simulink library "wcdma_lib"  (Simulink 6.0)
settings: Solver=ode45  SolverMode=SingleTasking  StartTime=0.0  StopTime=10.0  RelTol=1e-3
values from neighbouring files (symbols this model uses):
  allocationssc = [1 1 1 1 1 1 1 1 1 1 1 1 ... (960 elements, 64x15)]    [wcdma_allocationssc.mat]
  crcSize = str2num(Vals{idxCrcSize})    [wcdma_initmaskphlayer.m]    (also in wcdma_loadinitmuxandcoding.m = [16 12]; wcdma_loadinitphlayer.m = [16 12])
  errorCorr = (errorCorr>2)*2 + (errorCorr<3).*errorCorr    [wcdma_initmaskphlayer.m]    (also in wcdma_loadinitmuxandcoding.m = [2 2]; wcdma_loadinitphlayer.m = [2 2])
  i = [1:2:numSamp-1]'    [cdma2000_inttable.m]
  numBitsCodeWord = cond.*Zmin + not(cond).*numBitsCodeWord    [wcdma_concseg.m]    (also in wcdma_loadinitmuxandcoding.m = [260 122])
  numBitsFirstInt = numBitsRM + deltaNimax    [wcdma_initmaskphlayer.m]    (also in wcdma_loadinitmuxandcoding.m = [686 308])
  numBitsRF = numBitsFirstInt./(tti/10)    [wcdma_initmaskphlayer.m]    (also in wcdma_loadinitmuxandcoding.m = [343 77]; wcdma_loadinitphlayer.m = [343 77])
  numBitsTrCh = (trBlkSize+crcSize)*diag(numTrBlks)    [wcdma_concseg.m]    (also in wcdma_loadinitmuxandcoding.m = [260 112])
  numCodeWords = ceil(numBitsTrCh./Zmax(errorCorr+1))    [wcdma_concseg.m]    (also in wcdma_loadinitmuxandcoding.m = [1 1])
  numPadBits = (numBitsCodeWord.*numCodeWords)-numBitsTrCh    [wcdma_concseg.m]    (also in wcdma_loadinitmuxandcoding.m = [0 0])
  numPhCH = str2num(Vals{idxNumPhCH})    [wcdma_initmaskphlayer.m]    (also in wcdma_loadinitmuxandcoding.m = 1; wcdma_loadinitphlayer.m = 1)
  numTrBlks = trBlkSetSize./trBlkSize    [wcdma_concseg.m]    (also in wcdma_initmaskphlayer.m; wcdma_loadinitmuxandcoding.m = [1 1]; wcdma_loadinitphlayer.m = [1 1])
  overSampling = str2num(Vals{idxOverSampling})    [wcdma_initmaskphlayer.m]    (also in wcdma_initmaskspreadandmod.m; wcdma_loadinitphlayer.m = 8; wcdma_loadinitspreadandmod.m = 8)
  powerVector = str2num(Vals{idxPowerVector})    [wcdma_initmaskphlayer.m]    (also in wcdma_initmaskspreadandmod.m; wcdma_loadinitphlayer.m = [-5.5 -10 -15 -12 -12]; wcdma_loadinitspreadandmod.m = [-5.5 -10 -15 -12 -12])
  sprdFactor = wcdma_slotformattable(slotFormat+1,2)    [wcdma_checkparamstxant.m]    (also in wcdma_initmaskphlayer.m = slotformattable(slotFormat+1,2); wcdma_initmaskspreadandmod.m = slotformattable(slotFormat+1,2); wcdma_loadinitphlayer.m = 128; wcdma_loadinitspreadandmod.m = 128)
  tti = str2num(Vals{idxTti})    [wcdma_initmaskphlayer.m]    (also in wcdma_loadinitmuxandcoding.m = [20 40]; wcdma_loadinitphlayer.m = [20 40])
undefined symbols (not defined in the file or in its folder): hadamard, numSymbOut
libraries: wcdma_lib x122, dspsrcs4 x39, dspsigops x30, commseqgen2 x24, dspindex x20, dspbuff3 x19, dspmathops x16, simulink x10, dspsigattribs x7, commutil2 x6, dspmtrx3 x6, commblkintrlv2 x6
(part 3 of 3)

== system wcdma_lib/Wcdma Multiplexing and Channel Coding/Wcdma Tx  Channel Coding Scheme ==
  note: Wcdma Physical Channel TX Error Correction
  note: CRC
      | Calculation
  note: TrBlk Concat/
      | Code Blk Segm
  note: Channel
      | Coding
  note: 1st
      | Interleaver
  note: Rate
      | Matching
  note: Radio Frame
      | Segmentation
  TrChIn1 : Inport  LatchInput=off
  TrChIn2 : Inport  Port=2  LatchInput=off
  1st Interleaver : wcdma_lib/Wcdma Multiplexing and Channel Coding/1st Interleaver
  CRC Calculation : wcdma_lib/Wcdma Multiplexing and Channel Coding/CRC Calculation
  Channel Encoding : wcdma_lib/Wcdma Multiplexing and Channel Coding/Channel Encoding
  Radio Frame  Segmentation : wcdma_lib/Wcdma Multiplexing and Channel Coding/Radio Frame  Segmentation
  Rate Matching : wcdma_lib/Wcdma Multiplexing and Channel Coding/Rate Matching
  TrBlk Concatenat Code Blk Segment : wcdma_lib/Wcdma Multiplexing and Channel Coding/TrBlk Concatenat Code Blk Segment  numBitsTrCh=numBitsTrCh  numPadBits=numPadBits  numBitsCodeWord=numBitsCodeWord
  background6 : Subsystem  EnableExecutionContextPropagation=on
      mask Display: disp('')
  CCTrChOut1 : Outport
  wires:
  CRC Calculation/1 -> TrBlk Concatenat Code Blk Segment/1  "dtch"
  CRC Calculation/2 -> TrBlk Concatenat Code Blk Segment/2  "dcch"
  TrBlk Concatenat Code Blk Segment/1 -> Channel Encoding/1  "dtch"
  TrBlk Concatenat Code Blk Segment/2 -> Channel Encoding/2  "dcch"
  Channel Encoding/1 -> Rate Matching/1  "dtch"
  Channel Encoding/2 -> Rate Matching/2  "dcch"
  Rate Matching/1 -> 1st Interleaver/1  "dtch"
  Rate Matching/2 -> 1st Interleaver/2  "dcch"
  TrChIn1/1 -> CRC Calculation/1  "dtch"
  TrChIn2/1 -> CRC Calculation/2  "dcch"
  1st Interleaver/1 -> Radio Frame  Segmentation/1  "dtch"
  1st Interleaver/2 -> Radio Frame  Segmentation/2  "dcch"
  Radio Frame  Segmentation/1 -> CCTrChOut1/1  "cctrch"

== system wcdma_lib/Wcdma Sources/Channel Generator ==
  "Complex Unipolar to Bipolar " : wcdma_lib/Wcdma Common/Complex Unipolar to Bipolar   M=2  polarity=Negative
  Deinterlacer : commsequence2/Deinterlacer
  Delay : dspsigops/Delay  dly_unit=Samples  delay=initDelay  ic_detail=off  dif_ic_for_ch=off  dif_ic_for_dly=off  ic=0  reset_popup=None
  Gain : Gain  Gain=1/sqrt(2)  SaturateOnIntegerOverflow=on
  Random-Integer Generator : commrandsrc2/Random Integer Generator  mul=2  seed=rndSeed  Ts=st/2  frameBased=on  sampPerFrame=2*numSymbOut  orient=off
  Real-Imag to Complex : RealImagToComplex
  cChannel : Outport
  wires:
  Deinterlacer/2 -> Real-Imag to Complex/2
  Deinterlacer/1 -> Real-Imag to Complex/1
  "Complex Unipolar to Bipolar "/1 -> Gain/1
  Real-Imag to Complex/1 -> "Complex Unipolar to Bipolar "/1
  Gain/1 -> Delay/1
  Random-Integer Generator/1 -> Deinterlacer/1
  Delay/1 -> cChannel/1

== system wcdma_lib/Wcdma Sources/P-CPICH Generator ==
  "Complex Unipolar to Bipolar " : wcdma_lib/Wcdma Common/Complex Unipolar to Bipolar   M=2  polarity=Negative
  DSP Constant : dspsrcs4/DSP Constant  Value=ones(2*numSymbOut,1)  InterpretAs1D=off  SampleMode=Discrete  Ts=numSymbOut*st  FramebasedOutput=on
  Deinterlacer : commsequence2/Deinterlacer
  Gain : Gain  Gain=1/sqrt(2)  SaturateOnIntegerOverflow=on
  Real-Imag to Complex : RealImagToComplex
  cP-CPICH : Outport
  wires:
  Gain/1 -> cP-CPICH/1
  "Complex Unipolar to Bipolar "/1 -> Gain/1
  DSP Constant/1 -> Deinterlacer/1
  Deinterlacer/1 -> Real-Imag to Complex/1
  Deinterlacer/2 -> Real-Imag to Complex/2
  Real-Imag to Complex/1 -> "Complex Unipolar to Bipolar "/1

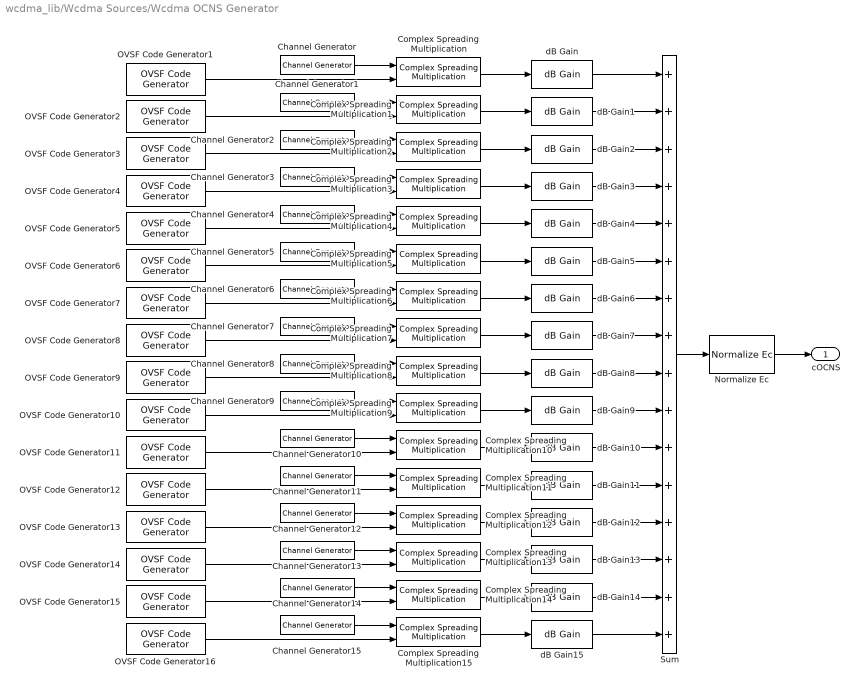
== system wcdma_lib/Wcdma Sources/Wcdma OCNS Generator ==
  Channel Generator : wcdma_lib/Wcdma Sources/Channel Generator  rndSeed=8686  initDelay=86  numSymbOut=numSymbOut  st=1/15e3
  Channel Generator1 : wcdma_lib/Wcdma Sources/Channel Generator  rndSeed=134134  initDelay=134  numSymbOut=numSymbOut  st=1/15e3
  Channel Generator10 : wcdma_lib/Wcdma Sources/Channel Generator  rndSeed=3030  initDelay=30  numSymbOut=numSymbOut  st=1/15e3
  Channel Generator11 : wcdma_lib/Wcdma Sources/Channel Generator  rndSeed=1818  initDelay=18  numSymbOut=numSymbOut  st=1/15e3
  Channel Generator12 : wcdma_lib/Wcdma Sources/Channel Generator  rndSeed=3030  initDelay=30  numSymbOut=numSymbOut  st=1/15e3
  Channel Generator13 : wcdma_lib/Wcdma Sources/Channel Generator  rndSeed=6161  initDelay=61  numSymbOut=numSymbOut  st=1/15e3
  Channel Generator14 : wcdma_lib/Wcdma Sources/Channel Generator  rndSeed=128128  initDelay=128  numSymbOut=numSymbOut  st=1/15e3
  Channel Generator15 : wcdma_lib/Wcdma Sources/Channel Generator  rndSeed=143143  initDelay=143  numSymbOut=numSymbOut  st=1/15e3
  Channel Generator2 : wcdma_lib/Wcdma Sources/Channel Generator  rndSeed=5252  initDelay=52  numSymbOut=numSymbOut  st=1/15e3
  Channel Generator3 : wcdma_lib/Wcdma Sources/Channel Generator  rndSeed=4545  initDelay=45  numSymbOut=numSymbOut  st=1/15e3
  Channel Generator4 : wcdma_lib/Wcdma Sources/Channel Generator  rndSeed=143143  initDelay=143  numSymbOut=numSymbOut  st=1/15e3
  Channel Generator5 : wcdma_lib/Wcdma Sources/Channel Generator  rndSeed=112112  initDelay=112  numSymbOut=numSymbOut  st=1/15e3
  Channel Generator6 : wcdma_lib/Wcdma Sources/Channel Generator  rndSeed=5959  initDelay=59  numSymbOut=numSymbOut  st=1/15e3
  Channel Generator7 : wcdma_lib/Wcdma Sources/Channel Generator  rndSeed=2323  initDelay=23  numSymbOut=numSymbOut  st=1/15e3
  Channel Generator8 : wcdma_lib/Wcdma Sources/Channel Generator  rndSeed=11  initDelay=1  numSymbOut=numSymbOut  st=1/15e3
  Channel Generator9 : wcdma_lib/Wcdma Sources/Channel Generator  rndSeed=8888  initDelay=88  numSymbOut=numSymbOut  st=1/15e3
  Complex Spreading Multiplication{,1..15} (16 alike) : wcdma_lib/Wcdma BS Transmitter/Complex Spreading Multiplication  sprdFactor=sprdFactor
  Normalize Ec : wcdma_lib/Wcdma Common/Normalize Ec
  OVSF Code Generator1 : commseqgen2/OVSF Code Generator  spreadFact=256  index=2  ts=1/15e3  frameBased=on  sampPerFrame=numChipsOut
  OVSF Code Generator10 : commseqgen2/OVSF Code Generator  spreadFact=256  index=69  ts=1/15e3  frameBased=on  sampPerFrame=numChipsOut
  OVSF Code Generator11 : commseqgen2/OVSF Code Generator  spreadFact=256  index=78  ts=1/15e3  frameBased=on  sampPerFrame=numChipsOut
  OVSF Code Generator12 : commseqgen2/OVSF Code Generator  spreadFact=256  index=85  ts=1/15e3  frameBased=on  sampPerFrame=numChipsOut
  OVSF Code Generator13 : commseqgen2/OVSF Code Generator  spreadFact=256  index=94  ts=1/15e3  frameBased=on  sampPerFrame=numChipsOut
  OVSF Code Generator14 : commseqgen2/OVSF Code Generator  spreadFact=256  index=125  ts=1/15e3  frameBased=on  sampPerFrame=numChipsOut
  OVSF Code Generator15 : commseqgen2/OVSF Code Generator  spreadFact=256  index=113  ts=1/15e3  frameBased=on  sampPerFrame=numChipsOut
  OVSF Code Generator16 : commseqgen2/OVSF Code Generator  spreadFact=256  index=119  ts=1/15e3  frameBased=on  sampPerFrame=numChipsOut
  OVSF Code Generator2 : commseqgen2/OVSF Code Generator  spreadFact=256  index=11  ts=1/15e3  frameBased=on  sampPerFrame=numChipsOut
  OVSF Code Generator3 : commseqgen2/OVSF Code Generator  spreadFact=256  index=17  ts=1/15e3  frameBased=on  sampPerFrame=numChipsOut
  OVSF Code Generator4 : commseqgen2/OVSF Code Generator  spreadFact=256  index=23  ts=1/15e3  frameBased=on  sampPerFrame=numChipsOut
  OVSF Code Generator5 : commseqgen2/OVSF Code Generator  spreadFact=256  index=31  ts=1/15e3  frameBased=on  sampPerFrame=numChipsOut
  OVSF Code Generator6 : commseqgen2/OVSF Code Generator  spreadFact=256  index=38  ts=1/15e3  frameBased=on  sampPerFrame=numChipsOut
  OVSF Code Generator7 : commseqgen2/OVSF Code Generator  spreadFact=256  index=47  ts=1/15e3  frameBased=on  sampPerFrame=numChipsOut
  OVSF Code Generator8 : commseqgen2/OVSF Code Generator  spreadFact=256  index=55  ts=1/15e3  frameBased=on  sampPerFrame=numChipsOut
  OVSF Code Generator9 : commseqgen2/OVSF Code Generator  spreadFact=256  index=62  ts=1/15e3  frameBased=on  sampPerFrame=numChipsOut
  Sum : Sum  Inputs=++++++++++++++++  SaturateOnIntegerOverflow=on  InputSameDT=on
  dB Gain : dspmathops/dB Gain  dB=-1  intype=Amplitude
  dB Gain1 : dspmathops/dB Gain  dB=-3  intype=Amplitude
  dB Gain10 : dspmathops/dB Gain  dB=-5  intype=Amplitude
  dB Gain11 : dspmathops/dB Gain  dB=-9  intype=Amplitude
  dB Gain12 : dspmathops/dB Gain  dB=-10  intype=Amplitude
  dB Gain13 : dspmathops/dB Gain  dB=-8  intype=Amplitude
  dB Gain14 : dspmathops/dB Gain  dB=-6  intype=Amplitude
  dB Gain15 : dspmathops/dB Gain  dB=0  intype=Amplitude
  dB Gain2 : dspmathops/dB Gain  dB=-3  intype=Amplitude
  dB Gain3 : dspmathops/dB Gain  dB=-5  intype=Amplitude
  dB Gain4 : dspmathops/dB Gain  dB=-2  intype=Amplitude
  dB Gain5 : dspmathops/dB Gain  dB=-4  intype=Amplitude
  dB Gain6 : dspmathops/dB Gain  dB=-8  intype=Amplitude
  dB Gain7 : dspmathops/dB Gain  dB=-7  intype=Amplitude
  dB Gain8 : dspmathops/dB Gain  dB=-4  intype=Amplitude
  dB Gain9 : dspmathops/dB Gain  dB=-6  intype=Amplitude
  cOCNS : Outport
  wires:
  Channel Generator/1 -> Complex Spreading Multiplication/1
  Channel Generator1/1 -> Complex Spreading Multiplication1/1
  Channel Generator2/1 -> Complex Spreading Multiplication2/1
  Channel Generator3/1 -> Complex Spreading Multiplication3/1
  Channel Generator4/1 -> Complex Spreading Multiplication4/1
  Channel Generator5/1 -> Complex Spreading Multiplication5/1
  Channel Generator6/1 -> Complex Spreading Multiplication6/1
  Channel Generator7/1 -> Complex Spreading Multiplication7/1
  Channel Generator8/1 -> Complex Spreading Multiplication8/1
  Channel Generator9/1 -> Complex Spreading Multiplication9/1
  Channel Generator10/1 -> Complex Spreading Multiplication10/1
  Channel Generator11/1 -> Complex Spreading Multiplication11/1
  Channel Generator12/1 -> Complex Spreading Multiplication12/1
  Channel Generator13/1 -> Complex Spreading Multiplication13/1
  Channel Generator14/1 -> Complex Spreading Multiplication14/1
  Channel Generator15/1 -> Complex Spreading Multiplication15/1
  OVSF Code Generator16/1 -> Complex Spreading Multiplication15/2
  OVSF Code Generator1/1 -> Complex Spreading Multiplication/2
  OVSF Code Generator2/1 -> Complex Spreading Multiplication1/2
  OVSF Code Generator3/1 -> Complex Spreading Multiplication2/2
  OVSF Code Generator4/1 -> Complex Spreading Multiplication3/2
  OVSF Code Generator5/1 -> Complex Spreading Multiplication4/2
  OVSF Code Generator6/1 -> Complex Spreading Multiplication5/2
  OVSF Code Generator7/1 -> Complex Spreading Multiplication6/2
  OVSF Code Generator8/1 -> Complex Spreading Multiplication7/2
  OVSF Code Generator9/1 -> Complex Spreading Multiplication8/2
  OVSF Code Generator10/1 -> Complex Spreading Multiplication9/2
  OVSF Code Generator11/1 -> Complex Spreading Multiplication10/2
  OVSF Code Generator12/1 -> Complex Spreading Multiplication11/2
  OVSF Code Generator13/1 -> Complex Spreading Multiplication12/2
  OVSF Code Generator14/1 -> Complex Spreading Multiplication13/2
  OVSF Code Generator15/1 -> Complex Spreading Multiplication14/2
  Complex Spreading Multiplication1/1 -> dB Gain1/1
  Complex Spreading Multiplication2/1 -> dB Gain2/1
  Complex Spreading Multiplication3/1 -> dB Gain3/1
  Complex Spreading Multiplication4/1 -> dB Gain4/1
  Complex Spreading Multiplication5/1 -> dB Gain5/1
  Complex Spreading Multiplication6/1 -> dB Gain6/1
  Complex Spreading Multiplication7/1 -> dB Gain7/1
  Complex Spreading Multiplication8/1 -> dB Gain8/1
  Complex Spreading Multiplication9/1 -> dB Gain9/1
  Complex Spreading Multiplication10/1 -> dB Gain10/1
  Complex Spreading Multiplication11/1 -> dB Gain11/1
  Complex Spreading Multiplication12/1 -> dB Gain12/1
  Complex Spreading Multiplication13/1 -> dB Gain13/1
  Complex Spreading Multiplication14/1 -> dB Gain14/1
  Complex Spreading Multiplication15/1 -> dB Gain15/1
  Sum/1 -> Normalize Ec/1
  dB Gain/1 -> Sum/1
  dB Gain1/1 -> Sum/2
  dB Gain2/1 -> Sum/3
  dB Gain3/1 -> Sum/4
  dB Gain4/1 -> Sum/5
  dB Gain5/1 -> Sum/6
  dB Gain6/1 -> Sum/7
  dB Gain7/1 -> Sum/8
  dB Gain8/1 -> Sum/9
  dB Gain9/1 -> Sum/10
  dB Gain10/1 -> Sum/11
  dB Gain11/1 -> Sum/12
  dB Gain12/1 -> Sum/13
  dB Gain13/1 -> Sum/14
  dB Gain14/1 -> Sum/15
  dB Gain15/1 -> Sum/16
  Complex Spreading Multiplication/1 -> dB Gain/1
  Normalize Ec/1 -> cOCNS/1

== system wcdma_lib/Wcdma Sources/Wcdma PSC Generator ==
  Frame Status Conversion : dspsigattribs/Frame Status Conversion  growRefPort=off  outframe=Frame-based
  Gain1 : Gain  Gain=1/sqrt(2)  SaturateOnIntegerOverflow=on
  Matrix Multiply : dspmtrx3/Matrix Multiply  numInputPorts=2  OptimizationLevel=None
  Pattern Repetition : dspsrcs4/DSP Constant  Value="[1 1 1 -1 -1 1 -1 -1  1 1 1 -1 1 -1 1 1]"  InterpretAs1D=off  SampleMode=Discrete  Ts=0.01/15  FramebasedOutput=on
  Real-Imag to Complex : RealImagToComplex
  Reshape : simulink3/Signals & Systems/Reshape  OutputDimensionality=Column vector  OutputDimensions=[1,1]
  Seq a : dspsrcs4/DSP Constant  Value=[1 1 1 1 1 1 -1 -1 1 -1 1 -1 1 -1 -1 1]'  InterpretAs1D=off  SampleMode=Discrete  Ts=0.01/15  FramebasedOutput=on
  PSC Code : Outport
  wires:
  Gain1/1 -> PSC Code/1
  Seq a/1 -> Matrix Multiply/1
  Pattern Repetition/1 -> Matrix Multiply/2
  Matrix Multiply/1 -> Reshape/1
  Real-Imag to Complex/1 -> Gain1/1
  Reshape/1 -> Frame Status Conversion/1
  Frame Status Conversion/1 -> Real-Imag to Complex/1, Real-Imag to Complex/2

== system wcdma_lib/Wcdma Sources/Wcdma Pilot Bits Generator ==
  Frame Status Conversion : dspsigattribs/Frame Status Conversion  growRefPort=off  outframe=Frame-based
  Integer to Bit Converter : commutil2/Integer to Bit Converter  nbits=numPilotBits
  Pilot Bits Generator : dspsrcs4/Signal From Workspace  X=pilotBits  Ts=0.01/15  nsamps=1  OutputAfterFinalValue=Cyclic Repetition
  PilotBitsOut : Outport
  wires:
  Pilot Bits Generator/1 -> Integer to Bit Converter/1
  Integer to Bit Converter/1 -> Frame Status Conversion/1
  Frame Status Conversion/1 -> PilotBitsOut/1

== system wcdma_lib/Wcdma Sources/Wcdma SCH  Generator ==
  Gain1 : Gain  Gain=1/sqrt(2)  SaturateOnIntegerOverflow=on
  Sum : Sum  SaturateOnIntegerOverflow=on  InputSameDT=on
  Wcdma PSC Generator : wcdma_lib/Wcdma Sources/Wcdma PSC Generator  a_sch=a_sch
  Wcdma SSC Generator : wcdma_lib/Wcdma Sources/Wcdma SSC Generator  scrGroup=scrGroup  a_sch=a_sch
  cSCH : Outport
  wires:
  Gain1/1 -> cSCH/1
  Wcdma PSC Generator/1 -> Sum/1
  Wcdma SSC Generator/1 -> Sum/2
  Sum/1 -> Gain1/1

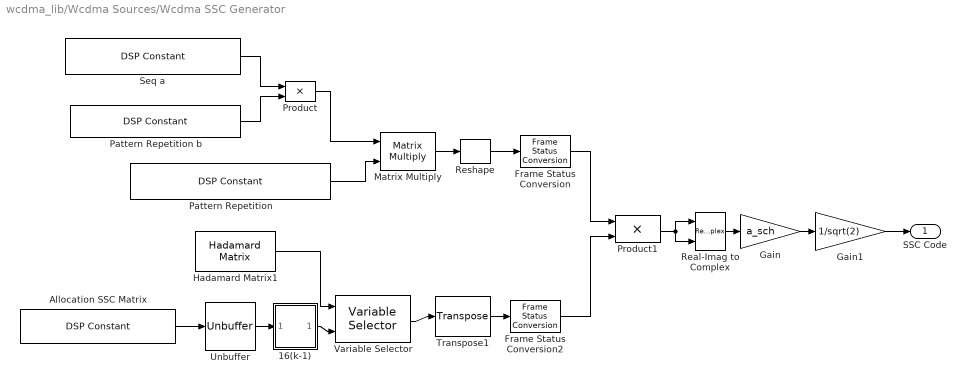
== system wcdma_lib/Wcdma Sources/Wcdma SSC Generator ==
  16(k-1) : Subsystem  EnableExecutionContextPropagation=on
      mask Display: disp('16(K-1)');
  Allocation SSC Matrix : dspsrcs4/DSP Constant  Value=allocationssc(scrGroup+1,:)'  InterpretAs1D=off  SampleMode=Discrete  Ts=0.01  FramebasedOutput=on
  Frame Status Conversion : dspsigattribs/Frame Status Conversion  growRefPort=off  outframe=Frame-based
  Frame Status Conversion2 : dspsigattribs/Frame Status Conversion  growRefPort=off  outframe=Frame-based
  Gain : Gain  Gain=a_sch  SaturateOnIntegerOverflow=on
  Gain1 : Gain  Gain=1/sqrt(2)  SaturateOnIntegerOverflow=on
  Hadamard Matrix1 : wcdma_lib/Wcdma Common/Hadamard Matrix  order=8
  Matrix Multiply : dspmtrx3/Matrix Multiply  numInputPorts=2  OptimizationLevel=None
  Pattern Repetition : dspsrcs4/DSP Constant  Value="[1 1 1 -1 -1 1 -1 -1  1 1 1 -1 1 -1 1 1]"  InterpretAs1D=off  SampleMode=Discrete  Ts=0.01/15  FramebasedOutput=on
  Pattern Repetition b : dspsrcs4/DSP Constant  Value=[ones(8,1) ; -1*ones(8,1)]  InterpretAs1D=off  SampleMode=Discrete  Ts=0.01/15  FramebasedOutput=on
  Product : Product  SaturateOnIntegerOverflow=on  InputSameDT=on
  Product1 : Product  SaturateOnIntegerOverflow=on  InputSameDT=on
  Real-Imag to Complex : RealImagToComplex
  Reshape : simulink3/Signals & Systems/Reshape  OutputDimensionality=Column vector  OutputDimensions=[1,1]
  Seq a : dspsrcs4/DSP Constant  Value=[1 1 1 1 1 1 -1 -1 1 -1 1 -1 1 -1 -1 1]'  InterpretAs1D=off  SampleMode=Discrete  Ts=0.01/15  FramebasedOutput=on
  Transpose1 : dspmtrx3/Transpose  Hermitian=off
  Unbuffer : dspbuff3/Unbuffer  ic=0
  Variable Selector : dspindex/Variable Selector  rowsOrCols=Rows  IdxMode=Variable  Elements=[1 3]  errmode=Clip and Warn
  SSC Code : Outport
  wires:
  Gain1/1 -> SSC Code/1
  Pattern Repetition/1 -> Matrix Multiply/2
  Matrix Multiply/1 -> Reshape/1
  Reshape/1 -> Frame Status Conversion/1
  Pattern Repetition b/1 -> Product/2
  Seq a/1 -> Product/1
  Product/1 -> Matrix Multiply/1
  Hadamard Matrix1/1 -> Variable Selector/1
  Unbuffer/1 -> 16(k-1)/1(In1)
  16(k-1)/1(Out1) -> Variable Selector/2
  Allocation SSC Matrix/1 -> Unbuffer/1
  Variable Selector/1 -> Transpose1/1
  Transpose1/1 -> Frame Status Conversion2/1
  Real-Imag to Complex/1 -> Gain/1
  Frame Status Conversion2/1 -> Product1/2
  Frame Status Conversion/1 -> Product1/1
  Product1/1 -> Real-Imag to Complex/1, Real-Imag to Complex/2
  Gain/1 -> Gain1/1

== system wcdma_lib/Wcdma Sources/Wcdma Scrambling Code Generator ==
  Gain : Gain  Gain=1/sqrt(2)  SaturateOnIntegerOverflow=on
  Gold Sequence Generator : commseqgen2/Gold Sequence Generator  genPoly1=[18 10 7 5 0]  iniState1=1  genPoly2=[18 7 0]  iniState2=[zeros(1,17) 1]  index=16*8*scrCode(1)+16*scrCode(2)  shift=0  ts=1/3.84e6  frameBased=on  sampPerFrame=numChipsOut  reset=on
  Gold Sequence Generator1 : commseqgen2/Gold Sequence Generator  genPoly1=[18 10 7 5 0]  iniState1=1  genPoly2=[18 7 0]  iniState2=[zeros(1,17) 1]  index=16*8*scrCode(1)+16*scrCode(2)  shift=131072  ts=1/3.84e6  frameBased=on  sampPerFrame=numChipsOut  reset=on
  Pulse Generator : DiscretePulseGenerator  Period=150/(numChipsOut/256)  SampleTime=(numChipsOut/256)/15e3
  Real-Imag to Complex : RealImagToComplex
  Unipolar to Bipolar Converter1 : commutil2/Unipolar to Bipolar Converter  M=2  polarity=Negative
  Unipolar to Bipolar Converter2 : commutil2/Unipolar to Bipolar Converter  M=2  polarity=Negative
  background1 : Subsystem  EnableExecutionContextPropagation=on
      mask Display: disp('')
  background2 : Subsystem  EnableExecutionContextPropagation=on
      mask Display: disp('')
  cScr_Code : Outport
  wires:
  Real-Imag to Complex/1 -> Gain/1
  Gain/1 -> cScr_Code/1  "Scrambling Code"
  Pulse Generator/1 -> Gold Sequence Generator/1, Gold Sequence Generator1/1  "Reset"
  Gold Sequence Generator/1 -> Unipolar to Bipolar Converter1/1  "Zn"
  Unipolar to Bipolar Converter1/1 -> Real-Imag to Complex/1  "Real Part"
  Unipolar to Bipolar Converter2/1 -> Real-Imag to Complex/2  "Imag Part"
  Gold Sequence Generator1/1 -> Unipolar to Bipolar Converter2/1  "Zn'"

== system wcdma_lib/Wcdma UE Receiver/I&Q Demapping ==
  In1 : Inport  LatchInput=off
  Complex to Real-Imag : ComplexToRealImag
  Interlacer : commsequence2/Interlacer
  Out1 : Outport
  wires:
  In1/1 -> Complex to Real-Imag/1
  Interlacer/1 -> Out1/1
  Complex to Real-Imag/2 -> Interlacer/2
  Complex to Real-Imag/1 -> Interlacer/1

== system wcdma_lib/Wcdma UE Receiver/Slot Rebuilder ==
  BitsIn : Inport  LatchInput=off
  Buffer : dspbuff3/Buffer  N=numBits  V=0  ic=0
  Delay : dspsigops/Delay  dly_unit=Samples  delay=numBits-mod(totalDelay,numBits)  ic_detail=off  dif_ic_for_ch=off  dif_ic_for_dly=off  ic=0  reset_popup=None
  SlotOut : Outport
  wires:
  Delay/1 -> Buffer/1
  Buffer/1 -> SlotOut/1  "Slots"
  BitsIn/1 -> Delay/1  "Bits"

== system wcdma_lib/Wcdma UE Receiver/Wcdma Channel Estimation ==
  cPICH Ref : Inport  LatchInput=off
  cPICH Rx : Inport  Port=2  LatchInput=off
  Finger Phase : Inport  Port=3  LatchInput=off
  Gain : Gain  Gain=1/sqrt(2)  SaturateOnIntegerOverflow=on
  Low Pass Filter : wcdma_lib/Wcdma Common/Low Pass Filter  N=(numTapsChEst-1)*(numChipsOut/256)  Wn=1/4  outputBufInitCond=0
  Math Function : Math  Operator=conj  OutputSignalType=complex  SaturateOnIntegerOverflow=on
  Product : Product  SaturateOnIntegerOverflow=on  InputSameDT=on
  Variable Integer Delay : dspsigops/Variable Integer Delay  dmax=1000  ic=0
  chEstimate : Outport
  wires:
  Finger Phase/1 -> Variable Integer Delay/2
  Variable Integer Delay/1 -> Math Function/1  "PICH Reference"
  cPICH Ref/1 -> Gain/1
  Math Function/1 -> Product/1
  Product/1 -> Low Pass Filter/1  "noisy channel estimate"
  cPICH Rx/1 -> Product/2  "Output of  Pilot Correlator"
  Gain/1 -> Variable Integer Delay/1
  Low Pass Filter/1 -> chEstimate/1

== system wcdma_lib/Wcdma UE Receiver/Wcdma Correlator ==
  cIn : Inport  LatchInput=off
  cPNseq : Inport  Port=2  LatchInput=off
  Enable : EnablePort
  Integrate and Dump : commfilt2/Integrate and Dump  obssamples=sprdFactor  offsetsamples=0  nodump=off
  Math Function : Math  Operator=conj  OutputSignalType=complex  SaturateOnIntegerOverflow=on
  Normalization : Gain  Gain=1/sprdFactor  SaturateOnIntegerOverflow=on
  Product2 : Product  Inputs=**  SaturateOnIntegerOverflow=on  InputSameDT=on
  Out1 : Outport
  wires:
  Math Function/1 -> Product2/2
  cPNseq/1 -> Math Function/1  "Chips Code"
  cIn/1 -> Product2/1  "Chips Signal"
  Product2/1 -> Integrate and Dump/1
  Integrate and Dump/1 -> Normalization/1
  Normalization/1 -> Out1/1

== system wcdma_lib/Wcdma UE Receiver/Wcdma Data Derotation ==
  cChEst : Inport  LatchInput=off
  cData_In : Inport  Port=2  LatchInput=off
  Math Function : Math  Operator=conj  SaturateOnIntegerOverflow=on
  Mean : dspstat3/Mean  run=off  reset_popup=None
  Product : Product  SaturateOnIntegerOverflow=on  InputSameDT=on
  cData_Out : Outport
  wires:
  Math Function/1 -> Product/1
  cChEst/1 -> Mean/1
  Product/1 -> cData_Out/1
  cData_In/1 -> Product/2
  Mean/1 -> Math Function/1

== system wcdma_lib/Wcdma UE Receiver/Wcdma Orthogonal  Codes Generator ==
  OVSF Code Generator : commseqgen2/OVSF Code Generator  spreadFact=256  index=0  ts=st  frameBased=on  sampPerFrame=numChipsOut
  OVSF Code Generator1 : commseqgen2/OVSF Code Generator  spreadFact=sprdFactor  index=codeNumber  ts=st  frameBased=on  sampPerFrame=numChipsOut
  Product1 : Product  Inputs=**  SaturateOnIntegerOverflow=on  InputSameDT=on
  Product2 : Product  Inputs=**  SaturateOnIntegerOverflow=on  InputSameDT=on
  Wcdma Scrambling Code Generator : wcdma_lib/Wcdma Sources/Wcdma Scrambling Code Generator  scrCode=scrCode  chipRate=3.84e6  numChipsOut=numChipsOut
  cPN_CPICH : Outport
  cPN_DPCH : Outport  Port=2
  wires:
  OVSF Code Generator/1 -> Product2/1  "OVSF CPICH"
  Wcdma Scrambling Code Generator/1 -> Product2/2, Product1/1  "Scr Code"
  OVSF Code Generator1/1 -> Product1/2  "OVSF DPCH"
  Product2/1 -> cPN_CPICH/1
  Product1/1 -> cPN_DPCH/1

== system wcdma_lib/Wcdma UE Receiver/Wcdma Rake Combiner ==
  cDPCH1 : Inport  LatchInput=off
  cDPCH2 : Inport  Port=2  LatchInput=off
  cDPCH3 : Inport  Port=3  LatchInput=off
  cDPCH4 : Inport  Port=4  LatchInput=off
  Norm Factor : Inport  Port=5  LatchInput=off
  Enable : EnablePort
  Matrix Concatenation : simulink/Math Operations/Matrix Concatenation  numInports=4  catMethod=Horizontal
  Matrix Sum : dspmtrx3/Matrix Sum  Dim=Rows  roundingMode=Floor  overflowMode=off
  Product3 : Product  Inputs=*/  SaturateOnIntegerOverflow=on  InputSameDT=on
  Sum : Sum  Inputs=+  SaturateOnIntegerOverflow=on  InputSameDT=on
  cDPCH : Outport
  wires:
  Matrix Sum/1 -> Product3/1
  cDPCH4/1 -> Matrix Concatenation/4
  cDPCH3/1 -> Matrix Concatenation/3
  cDPCH2/1 -> Matrix Concatenation/2
  cDPCH1/1 -> Matrix Concatenation/1
  Matrix Concatenation/1 -> Matrix Sum/1
  Sum/1 -> Product3/2
  Norm Factor/1 -> Sum/1
  Product3/1 -> cDPCH/1

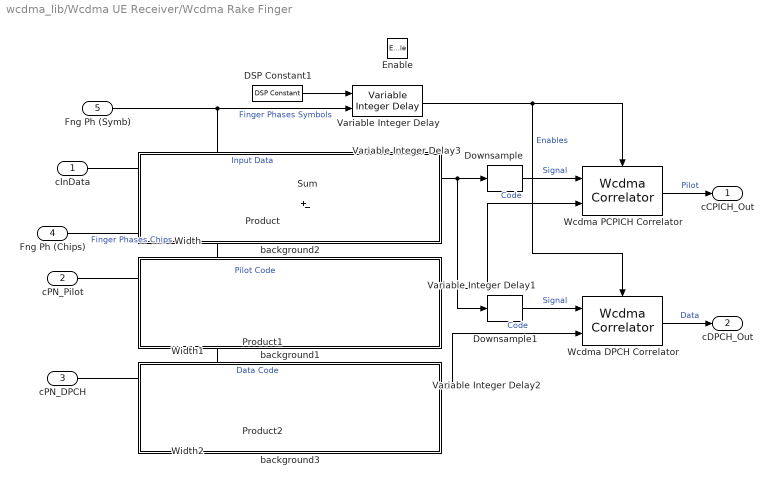
== system wcdma_lib/Wcdma UE Receiver/Wcdma Rake Finger ==
  cInData : Inport  LatchInput=off
  cPN_Pilot : Inport  Port=2  LatchInput=off
  cPN_DPCH : Inport  Port=3  LatchInput=off
  Fng Ph (Chips) : Inport  Port=4  LatchInput=off
  Fng Ph (Symb) : Inport  Port=5  LatchInput=off
  Enable : EnablePort
  DSP Constant1 : dspsrcs4/DSP Constant  Value=1  SampleMode=Discrete  discreteOutput=Sample-based  continuousOutput=Sample-based  sampTime=st  framePeriod=st  dataType=Inherit from 'Constant value'  wordLen=16  udDataType=sfix(16)  fracBitsMode=Best precision  numFracBits=15  InterpretAs1D=off  Ts=st  FramebasedOutput=off
  Downsample : dspsigops/Downsample  N=overSampling  phase=0  ic=0  smode=Force single rate  fmode=Maintain input frame rate
  Downsample1 : dspsigops/Downsample  N=overSampling  phase=0  ic=0  smode=Force single rate  fmode=Maintain input frame rate
  Product : Product  SaturateOnIntegerOverflow=on  InputSameDT=on
  Product1 : Product  SaturateOnIntegerOverflow=on  InputSameDT=on
  Product2 : Product  SaturateOnIntegerOverflow=on  InputSameDT=on
  Sum : Sum  Inputs=|+-  SaturateOnIntegerOverflow=on  InputSameDT=on
  Variable Integer Delay : dspsigops/Variable Integer Delay  dmax=100  ic=0
  Variable Integer Delay1 : dspsigops/Variable Integer Delay  dmax=100*256  ic=0
  Variable Integer Delay2 : dspsigops/Variable Integer Delay  dmax=100*256  ic=0
  Variable Integer Delay3 : dspsigops/Variable Integer Delay  dmax=100*256  ic=0
  Wcdma DPCH Correlator : wcdma_lib/Wcdma UE Receiver/Wcdma Correlator  sprdFactor=sprdFactor
  Wcdma PCPICH Correlator : wcdma_lib/Wcdma UE Receiver/Wcdma Correlator  sprdFactor=256
  Width : Width
  Width1 : Width
  Width2 : Width
  background1 : Subsystem  EnableExecutionContextPropagation=on
      mask Display: disp('')
  background2 : Subsystem  EnableExecutionContextPropagation=on
      mask Display: disp('')
  background3 : Subsystem  EnableExecutionContextPropagation=on
      mask Display: disp('')
  cCPICH_Out : Outport
  cDPCH_Out : Outport  Port=2
  wires:
  Variable Integer Delay2/1 -> Wcdma DPCH Correlator/2  "Code"
  Fng Ph (Chips)/1 -> Sum/2  "Finger Phases Chips"
  Sum/1 -> Variable Integer Delay3/2
  Product/1 -> Sum/1
  Width2/1 -> Product2/2
  Product2/1 -> Variable Integer Delay2/2
  cPN_DPCH/1 -> Variable Integer Delay2/1, Width2/1  "Data Code"
  Width1/1 -> Product1/2
  Width/1 -> Product/2
  Product1/1 -> Variable Integer Delay1/2
  Fng Ph (Symb)/1 -> Product/1, Product1/1, Product2/1, Variable Integer Delay/2  "Finger Phases Symbols"
  cInData/1 -> Width/1, Variable Integer Delay3/1  "Input Data"
  Variable Integer Delay3/1 -> Downsample1/1, Downsample/1
  Wcdma PCPICH Correlator/1 -> cCPICH_Out/1  "Pilot"
  Wcdma DPCH Correlator/1 -> cDPCH_Out/1  "Data"
  Variable Integer Delay/1 -> Wcdma DPCH Correlator/Enable, Wcdma PCPICH Correlator/Enable  "Enables"
  DSP Constant1/1 -> Variable Integer Delay/1
  Downsample/1 -> Wcdma PCPICH Correlator/1  "Signal"
  Downsample1/1 -> Wcdma DPCH Correlator/1  "Signal"
  cPN_Pilot/1 -> Width1/1, Variable Integer Delay1/1  "Pilot Code"
  Variable Integer Delay1/1 -> Wcdma PCPICH Correlator/2  "Code"

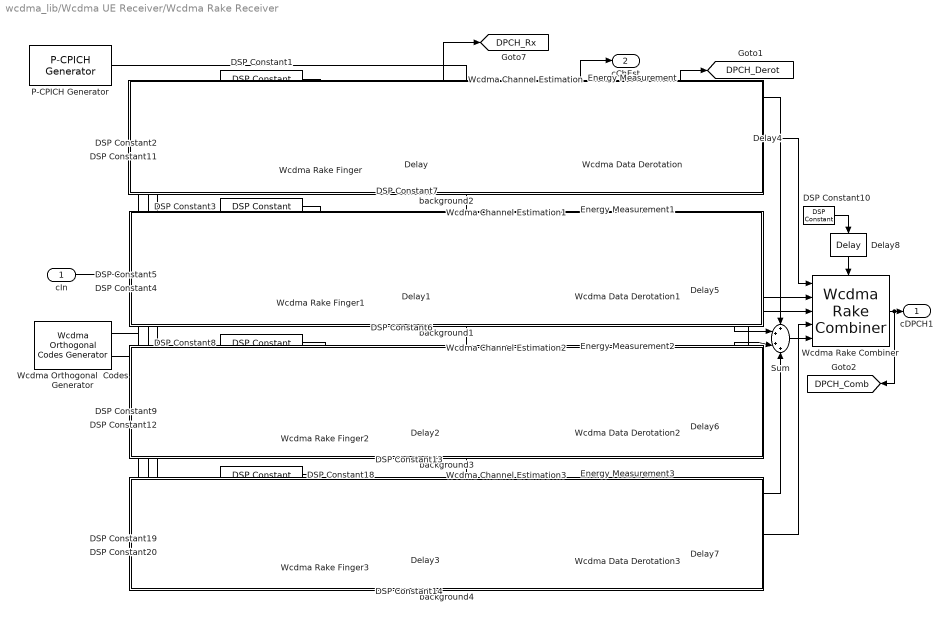
== system wcdma_lib/Wcdma UE Receiver/Wcdma Rake Receiver ==
  cIn : Inport  LatchInput=off
  DSP Constant1 : dspsrcs4/DSP Constant  Value=fingerEnables(1)  SampleMode=Discrete  discreteOutput=Sample-based  continuousOutput=Sample-based  sampTime=st  framePeriod=st  dataType=Inherit from 'Constant value'  wordLen=16  udDataType=sfix(16)  fracBitsMode=Best precision  numFracBits=15  InterpretAs1D=off  Ts=st  FramebasedOutput=off
  DSP Constant10 : dspsrcs4/DSP Constant  Value=1  SampleMode=Discrete  discreteOutput=Sample-based  continuousOutput=Sample-based  sampTime=st  framePeriod=st  dataType=Inherit from 'Constant value'  wordLen=16  udDataType=sfix(16)  fracBitsMode=Best precision  numFracBits=15  InterpretAs1D=off  Ts=st  FramebasedOutput=off
  DSP Constant11 : dspsrcs4/DSP Constant  Value=rxSymDelay(1)  SampleMode=Discrete  discreteOutput=Sample-based  continuousOutput=Sample-based  sampTime=st  framePeriod=st  dataType=Inherit from 'Constant value'  wordLen=16  udDataType=sfix(16)  fracBitsMode=Best precision  numFracBits=15  InterpretAs1D=off  Ts=st  FramebasedOutput=off
  DSP Constant12 : dspsrcs4/DSP Constant  Value=rxSymDelay(3)  SampleMode=Discrete  discreteOutput=Sample-based  continuousOutput=Sample-based  sampTime=st  framePeriod=st  dataType=Inherit from 'Constant value'  wordLen=16  udDataType=sfix(16)  fracBitsMode=Best precision  numFracBits=15  InterpretAs1D=off  Ts=st  FramebasedOutput=off
  DSP Constant13 : dspsrcs4/DSP Constant  Value=rxSymDelay(3)  SampleMode=Discrete  discreteOutput=Sample-based  continuousOutput=Sample-based  sampTime=st  framePeriod=st  dataType=Inherit from 'Constant value'  wordLen=16  udDataType=sfix(16)  fracBitsMode=Best precision  numFracBits=15  InterpretAs1D=off  Ts=st  FramebasedOutput=off
  DSP Constant14 : dspsrcs4/DSP Constant  Value=rxSymDelay(4)  SampleMode=Discrete  discreteOutput=Sample-based  continuousOutput=Sample-based  sampTime=st  framePeriod=st  dataType=Inherit from 'Constant value'  wordLen=16  udDataType=sfix(16)  fracBitsMode=Best precision  numFracBits=15  InterpretAs1D=off  Ts=st  FramebasedOutput=off
  DSP Constant18 : dspsrcs4/DSP Constant  Value=fingerEnables(4)  SampleMode=Discrete  discreteOutput=Sample-based  continuousOutput=Sample-based  sampTime=st  framePeriod=st  dataType=Inherit from 'Constant value'  wordLen=16  udDataType=sfix(16)  fracBitsMode=Best precision  numFracBits=15  InterpretAs1D=off  Ts=st  FramebasedOutput=off
  DSP Constant19 : dspsrcs4/DSP Constant  Value=rxTicksDelay(4)  SampleMode=Discrete  discreteOutput=Sample-based  continuousOutput=Sample-based  sampTime=st  framePeriod=st  dataType=Inherit from 'Constant value'  wordLen=16  udDataType=sfix(16)  fracBitsMode=Best precision  numFracBits=15  InterpretAs1D=off  Ts=st  FramebasedOutput=off
  DSP Constant2 : dspsrcs4/DSP Constant  Value=rxTicksDelay(1)  SampleMode=Discrete  discreteOutput=Sample-based  continuousOutput=Sample-based  sampTime=st  framePeriod=st  dataType=Inherit from 'Constant value'  wordLen=16  udDataType=sfix(16)  fracBitsMode=Best precision  numFracBits=15  InterpretAs1D=off  Ts=st  FramebasedOutput=off
  DSP Constant20 : dspsrcs4/DSP Constant  Value=rxSymDelay(4)  SampleMode=Discrete  discreteOutput=Sample-based  continuousOutput=Sample-based  sampTime=st  framePeriod=st  dataType=Inherit from 'Constant value'  wordLen=16  udDataType=sfix(16)  fracBitsMode=Best precision  numFracBits=15  InterpretAs1D=off  Ts=st  FramebasedOutput=off
  DSP Constant3 : dspsrcs4/DSP Constant  Value=fingerEnables(2)  SampleMode=Discrete  discreteOutput=Sample-based  continuousOutput=Sample-based  sampTime=st  framePeriod=st  dataType=Inherit from 'Constant value'  wordLen=16  udDataType=sfix(16)  fracBitsMode=Best precision  numFracBits=15  InterpretAs1D=off  Ts=st  FramebasedOutput=off
  DSP Constant4 : dspsrcs4/DSP Constant  Value=rxSymDelay(2)  SampleMode=Discrete  discreteOutput=Sample-based  continuousOutput=Sample-based  sampTime=st  framePeriod=st  dataType=Inherit from 'Constant value'  wordLen=16  udDataType=sfix(16)  fracBitsMode=Best precision  numFracBits=15  InterpretAs1D=off  Ts=st  FramebasedOutput=off
  DSP Constant5 : dspsrcs4/DSP Constant  Value=rxTicksDelay(2)  SampleMode=Discrete  discreteOutput=Sample-based  continuousOutput=Sample-based  sampTime=st  framePeriod=st  dataType=Inherit from 'Constant value'  wordLen=16  udDataType=sfix(16)  fracBitsMode=Best precision  numFracBits=15  InterpretAs1D=off  Ts=st  FramebasedOutput=off
  DSP Constant6 : dspsrcs4/DSP Constant  Value=rxSymDelay(2)  SampleMode=Discrete  discreteOutput=Sample-based  continuousOutput=Sample-based  sampTime=st  framePeriod=st  dataType=Inherit from 'Constant value'  wordLen=16  udDataType=sfix(16)  fracBitsMode=Best precision  numFracBits=15  InterpretAs1D=off  Ts=st  FramebasedOutput=off
  DSP Constant7 : dspsrcs4/DSP Constant  Value=rxSymDelay(1)  SampleMode=Discrete  discreteOutput=Sample-based  continuousOutput=Sample-based  sampTime=st  framePeriod=st  dataType=Inherit from 'Constant value'  wordLen=16  udDataType=sfix(16)  fracBitsMode=Best precision  numFracBits=15  InterpretAs1D=off  Ts=st  FramebasedOutput=off
  DSP Constant8 : dspsrcs4/DSP Constant  Value=fingerEnables(3)  SampleMode=Discrete  discreteOutput=Sample-based  continuousOutput=Sample-based  sampTime=st  framePeriod=st  dataType=Inherit from 'Constant value'  wordLen=16  udDataType=sfix(16)  fracBitsMode=Best precision  numFracBits=15  InterpretAs1D=off  Ts=st  FramebasedOutput=off
  DSP Constant9 : dspsrcs4/DSP Constant  Value=rxTicksDelay(3)  SampleMode=Discrete  discreteOutput=Sample-based  continuousOutput=Sample-based  sampTime=st  framePeriod=st  dataType=Inherit from 'Constant value'  wordLen=16  udDataType=sfix(16)  fracBitsMode=Best precision  numFracBits=15  InterpretAs1D=off  Ts=st  FramebasedOutput=off
  Delay{,1..3} (4 alike) : dspsigops/Delay  dly_unit=Samples  delay=((numTapsChEst-1)/2)*numSymbFrame  ic_detail=off  dif_ic_for_ch=off  dif_ic_for_dly=off  ic=0  reset_popup=None
  Delay4 : dspsigops/Delay  dly_unit=Samples  delay=(maxSymDelay-rxSymDelay(1))*numSymbFrame  ic_detail=off  dif_ic_for_ch=off  dif_ic_for_dly=off  ic=0  reset_popup=None
  Delay5 : dspsigops/Delay  dly_unit=Samples  delay=(maxSymDelay-rxSymDelay(2))*numSymbFrame  ic_detail=off  dif_ic_for_ch=off  dif_ic_for_dly=off  ic=0  reset_popup=None
  Delay6 : dspsigops/Delay  dly_unit=Samples  delay=(maxSymDelay-rxSymDelay(3))*numSymbFrame  ic_detail=off  dif_ic_for_ch=off  dif_ic_for_dly=off  ic=0  reset_popup=None
  Delay7 : dspsigops/Delay  dly_unit=Samples  delay=(maxSymDelay-rxSymDelay(4))*numSymbFrame  ic_detail=off  dif_ic_for_ch=off  dif_ic_for_dly=off  ic=0  reset_popup=None
  Delay8 : dspsigops/Delay  Orientation=down  dly_unit=Samples  delay=(((numTapsChEst-1)/2) +maxSymDelay)  ic_detail=off  dif_ic_for_ch=off  dif_ic_for_dly=off  ic=0  reset_popup=None
  Energy Measurement{,1..3} (4 alike) : wcdma_lib/Wcdma Common/Energy Measurement
  P-CPICH Generator : wcdma_lib/Wcdma Sources/P-CPICH Generator  antenna=1  numSymbOut=1  st=st
  Sum : Sum  Inputs=++++  SaturateOnIntegerOverflow=on  InputSameDT=on
  Wcdma Channel Estimation{,1..3} (4 alike) : wcdma_lib/Wcdma UE Receiver/Wcdma Channel Estimation  numTapsChEst=numTapsChEst  numChipsOut=numChipsOut
  Wcdma Data Derotation{,1..3} (4 alike) : wcdma_lib/Wcdma UE Receiver/Wcdma Data Derotation
  Wcdma Orthogonal  Codes Generator : wcdma_lib/Wcdma UE Receiver/Wcdma Orthogonal  Codes Generator  sprdFactor=sprdFactor  codeNumber=codeNumber  scrCode=scrCode  numChipsOut=numChipsOut  st=st
  Wcdma Rake Combiner : wcdma_lib/Wcdma UE Receiver/Wcdma Rake Combiner
  Wcdma Rake Finger{,1..3} (4 alike) : wcdma_lib/Wcdma UE Receiver/Wcdma Rake Finger  sprdFactor=sprdFactor  overSampling=overSampling  numChipsOut=numChipsOut  st=st
  background1 : Subsystem  EnableExecutionContextPropagation=on
      mask Display: disp('')
  background2 : Subsystem  EnableExecutionContextPropagation=on
      mask Display: disp('')
  background3 : Subsystem  EnableExecutionContextPropagation=on
      mask Display: disp('')
  background4 : Subsystem  EnableExecutionContextPropagation=on
      mask Display: disp('')
  cDPCH1 : Outport
  cChEst : Outport  Port=2
  tag scope: DPCH_Comb=global, DPCH_Derot=global, DPCH_Rx=global
  wires:
  Wcdma Rake Combiner/1 -> cDPCH1/1, [DPCH_Comb]
  Delay5/1 -> Wcdma Rake Combiner/2
  DSP Constant8/1 -> Wcdma Rake Finger2/Enable
  Wcdma Channel Estimation1/1 -> Wcdma Data Derotation1/1, Energy Measurement1/1
  Wcdma Rake Finger1/2 -> Delay1/1
  DSP Constant3/1 -> Wcdma Rake Finger1/Enable
  Wcdma Rake Finger1/1 -> Wcdma Channel Estimation1/2
  Wcdma Data Derotation1/1 -> Delay5/1
  Delay1/1 -> Wcdma Data Derotation1/2
  DSP Constant7/1 -> Wcdma Channel Estimation/3
  DSP Constant11/1 -> Wcdma Rake Finger/5
  Delay4/1 -> Wcdma Rake Combiner/1
  cIn/1 -> Wcdma Rake Finger/1, Wcdma Rake Finger1/1, Wcdma Rake Finger2/1, Wcdma Rake Finger3/1
  Wcdma Rake Finger/2 -> Delay/1
  DSP Constant2/1 -> Wcdma Rake Finger/4
  DSP Constant1/1 -> Wcdma Rake Finger/Enable
  Wcdma Orthogonal  Codes Generator/1 -> Wcdma Rake Finger1/2, Wcdma Rake Finger/2, Wcdma Rake Finger2/2, Wcdma Rake Finger3/2
  Wcdma Orthogonal  Codes Generator/2 -> Wcdma Rake Finger1/3, Wcdma Rake Finger/3, Wcdma Rake Finger2/3, Wcdma Rake Finger3/3
  P-CPICH Generator/1 -> Wcdma Channel Estimation/1, Wcdma Channel Estimation1/1, Wcdma Channel Estimation2/1, Wcdma Channel Estimation3/1
  Wcdma Rake Finger/1 -> Wcdma Channel Estimation/2
  Wcdma Data Derotation/1 -> [DPCH_Derot], Delay4/1
  Delay/1 -> Wcdma Data Derotation/2, [DPCH_Rx]
  Wcdma Channel Estimation/1 -> Wcdma Data Derotation/1, cChEst/1, Energy Measurement/1
  DSP Constant4/1 -> Wcdma Rake Finger1/5
  DSP Constant5/1 -> Wcdma Rake Finger1/4
  DSP Constant6/1 -> Wcdma Channel Estimation1/3
  DSP Constant9/1 -> Wcdma Rake Finger2/4
  DSP Constant12/1 -> Wcdma Rake Finger2/5
  Wcdma Rake Finger2/1 -> Wcdma Channel Estimation2/2
  DSP Constant13/1 -> Wcdma Channel Estimation2/3
  Wcdma Rake Finger2/2 -> Delay2/1
  Delay2/1 -> Wcdma Data Derotation2/2
  Wcdma Channel Estimation2/1 -> Wcdma Data Derotation2/1, Energy Measurement2/1
  Wcdma Data Derotation2/1 -> Delay6/1
  Delay6/1 -> Wcdma Rake Combiner/3
  DSP Constant18/1 -> Wcdma Rake Finger3/Enable
  DSP Constant19/1 -> Wcdma Rake Finger3/4
  DSP Constant20/1 -> Wcdma Rake Finger3/5
  Wcdma Rake Finger3/1 -> Wcdma Channel Estimation3/2
  DSP Constant14/1 -> Wcdma Channel Estimation3/3
  Wcdma Rake Finger3/2 -> Delay3/1
  Wcdma Channel Estimation3/1 -> Wcdma Data Derotation3/1, Energy Measurement3/1
  Delay3/1 -> Wcdma Data Derotation3/2
  Wcdma Data Derotation3/1 -> Delay7/1
  Delay7/1 -> Wcdma Rake Combiner/4
  Energy Measurement/1 -> Sum/1
  Sum/1 -> Wcdma Rake Combiner/5
  Energy Measurement1/1 -> Sum/2
  Energy Measurement2/1 -> Sum/3
  Energy Measurement3/1 -> Sum/4
  Delay8/1 -> Wcdma Rake Combiner/Enable
  DSP Constant10/1 -> Delay8/1

== system wcdma_lib/Wcdma UE Receiver/Wcdma UE Rx Antenna ==
  note: Wcdma UE Rx Antenna
  PhCHIn1 : Inport  LatchInput=off
  I&Q Demapping : wcdma_lib/Wcdma UE Receiver/I&Q Demapping
  Raised Cosine Receive Filter : commfilt2/Raised Cosine Receive Filter  filtType=Square root  N=overSampling  D=floor(numTapsRRC/(overSampling*2))  R=0.22  sampMode=Frame-based  rateMode=None  downFactor=8  downOffset=0  checkGain=User-specified  filterGain=1/sqrt(overSampling)  checkCoeff=off  variableName=rcRxFilt  launchFVT=off
  Slot Rebuilder : wcdma_lib/Wcdma UE Receiver/Slot Rebuilder  numBits=numBits  totalDelay=rxDelay*2
  Wcdma Rake Receiver : wcdma_lib/Wcdma UE Receiver/Wcdma Rake Receiver  sprdFactor=sprdFactor  codeNumber=dpchCode  scrCode=scrCode  numTapsChEst=numTapsChEst  numTapsRRC=numTapsRRC  overSampling=overSampling  fingerEnables=fingerEnables  fingerPhases=fingerPhases  numChipsOut=numChipsOut  st=1/15e3
  background2 : Subsystem  EnableExecutionContextPropagation=on
      mask Display: disp('')
  PhCHOut1 : Outport
  tag scope: RxSignal=global, chEst=global
  wires:
  I&Q Demapping/1 -> Slot Rebuilder/1  "dpch"
  Wcdma Rake Receiver/2 -> [chEst]  "chEst"
  Slot Rebuilder/1 -> PhCHOut1/1  "slot"
  Wcdma Rake Receiver/1 -> I&Q Demapping/1  "dpch"
  PhCHIn1/1 -> [RxSignal], Raised Cosine Receive Filter/1  "Rx Signal"
  Raised Cosine Receive Filter/1 -> Wcdma Rake Receiver/1

== system wcdma_lib/Wcdma BS Transmitter/Wcdma BS Tx Antenna/background1 ==

== system wcdma_lib/Wcdma BS Transmitter/Wcdma Spreading/background1 ==

== system wcdma_lib/Wcdma BS Transmitter/Wcdma Spreading/background2 ==

== system wcdma_lib/Wcdma Common/BLER Calculation/Combined BLER Calculation ==
  NumErrors1 : Inport  LatchInput=off
  NumErrors2 : Inport  Port=2  LatchInput=off
  NumBits1 : Inport  Port=3  LatchInput=off
  NumBits2 : Inport  Port=4  LatchInput=off
  Enable : EnablePort
  Matrix Concatenation : simulink/Math Operations/Matrix Concatenation  numInports=2  catMethod=Vertical
  Product : Product  Inputs=*/  SaturateOnIntegerOverflow=on  InputSameDT=on
  Sum : Sum  Inputs=|++  SaturateOnIntegerOverflow=on  InputSameDT=on
  Sum1 : Sum  Inputs=|++  SaturateOnIntegerOverflow=on  InputSameDT=on
  Zero-Order Hold : ZeroOrderHold  SampleTime=tti(i)*(1e-3)
  Zero-Order Hold1 : ZeroOrderHold  SampleTime=tti(i)*(1e-3)
  Combined BLER : Outport
  wires:
  Sum/1 -> Zero-Order Hold/1
  Product/1 -> Matrix Concatenation/1
  NumErrors1/1 -> Sum/1
  NumErrors2/1 -> Sum/2
  NumBits1/1 -> Sum1/1
  Matrix Concatenation/1 -> Combined BLER/1
  NumBits2/1 -> Sum1/2
  Zero-Order Hold/1 -> Product/1
  Sum1/1 -> Zero-Order Hold1/1
  Zero-Order Hold1/1 -> Matrix Concatenation/2, Product/2

== system wcdma_lib/Wcdma Common/Normalize Ec/Power  Measurement ==
  cIn : Inport  LatchInput=off
  Complex to Real-Imag : ComplexToRealImag
  Product : Product  SaturateOnIntegerOverflow=on  InputSameDT=on
  Product1 : Product  SaturateOnIntegerOverflow=on  InputSameDT=on
  Product2 : Product  Inputs=*/  SaturateOnIntegerOverflow=on  InputSameDT=on
  Sum1 : Sum  SaturateOnIntegerOverflow=on  InputSameDT=on
  Sum2 : Sum  Inputs=+  SaturateOnIntegerOverflow=on  InputSameDT=on
  Width : Width
  Power : Outport
  wires:
  Sum2/1 -> Product2/1
  Complex to Real-Imag/2 -> Product1/1, Product1/2
  Product2/1 -> Power/1
  Width/1 -> Product2/2
  Sum1/1 -> Sum2/1
  cIn/1 -> Width/1, Complex to Real-Imag/1
  Product/1 -> Sum1/1
  Product1/1 -> Sum1/2
  Complex to Real-Imag/1 -> Product/1, Product/2

== system wcdma_lib/Wcdma Multiplexing and Channel Coding/Wcdma Rx Channel Decoding Scheme/background6 ==

== system wcdma_lib/Wcdma Multiplexing and Channel Coding/Wcdma Rx PhCh Demapping/background6 ==

== system wcdma_lib/Wcdma Multiplexing and Channel Coding/Wcdma Tx PhCh Mapping/background6 ==

== system wcdma_lib/Wcdma Multiplexing and Channel Coding/Wcdma Tx  Channel Coding Scheme/background6 ==

== system wcdma_lib/Wcdma Sources/Wcdma SSC Generator/16(k-1) ==
  In1 : Inport  LatchInput=off
  DSP Constant : dspsrcs4/DSP Constant  Value=1  InterpretAs1D=off  SampleMode=Discrete  Ts=0.01/15  FramebasedOutput=on
  DSP Constant1 : dspsrcs4/DSP Constant  Value=1  InterpretAs1D=off  SampleMode=Discrete  Ts=0.01/15  FramebasedOutput=on
  Gain : Gain  Gain=16  SaturateOnIntegerOverflow=on
  Sum1 : Sum  Inputs=|++  SaturateOnIntegerOverflow=on  InputSameDT=on
  Sum2 : Sum  Inputs=|+-  SaturateOnIntegerOverflow=on  InputSameDT=on
  Out1 : Outport
  wires:
  Sum1/1 -> Out1/1
  DSP Constant1/1 -> Sum1/2
  DSP Constant/1 -> Sum2/2
  Gain/1 -> Sum1/1
  Sum2/1 -> Gain/1
  In1/1 -> Sum2/1

== system wcdma_lib/Wcdma Sources/Wcdma Scrambling Code Generator/background1 ==

== system wcdma_lib/Wcdma Sources/Wcdma Scrambling Code Generator/background2 ==

== system wcdma_lib/Wcdma UE Receiver/Wcdma Rake Finger/background1 ==

== system wcdma_lib/Wcdma UE Receiver/Wcdma Rake Finger/background2 ==

== system wcdma_lib/Wcdma UE Receiver/Wcdma Rake Finger/background3 ==

== system wcdma_lib/Wcdma UE Receiver/Wcdma Rake Receiver/background1 ==

== system wcdma_lib/Wcdma UE Receiver/Wcdma Rake Receiver/background2 ==

== system wcdma_lib/Wcdma UE Receiver/Wcdma Rake Receiver/background3 ==

== system wcdma_lib/Wcdma UE Receiver/Wcdma Rake Receiver/background4 ==

== system wcdma_lib/Wcdma UE Receiver/Wcdma UE Rx Antenna/background2 ==
